simulink model "Test1"  (R2018b)
settings: Solver=VariableStepAuto  StartTime=0.0  StopTime=10.0  MaxStep=0.002  MinStep=0.001  RelTol=1e-3
undefined symbols (not defined in the file or in its folder): sigbuilder_block
settings Model: Creator=wqq  LastModifiedBy=wqq
settings SolverCC: InitialStep=0.001

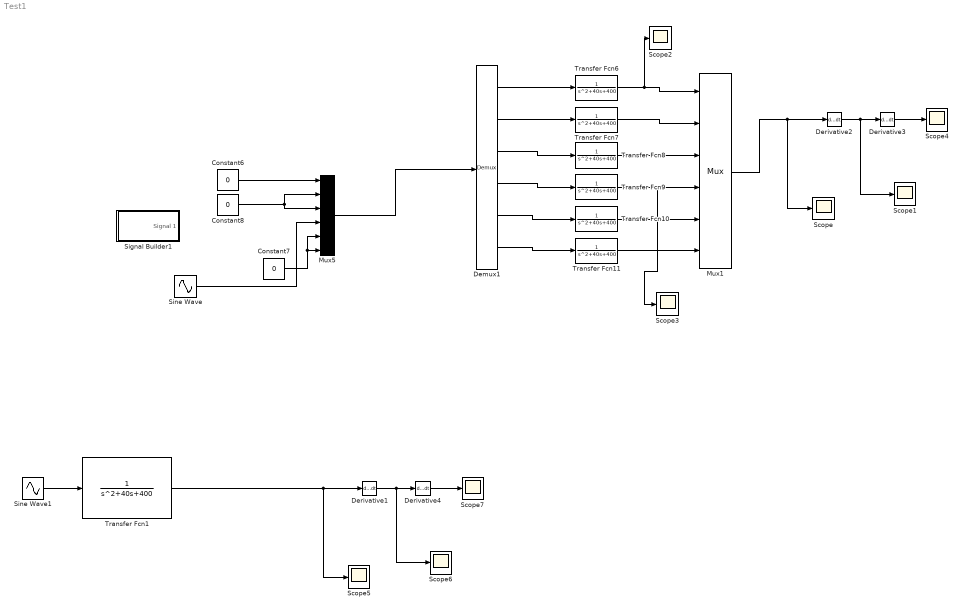
== system Test1 ==
  Constant6 : Constant  Value=0
  Constant7 : Constant  Value=0
  Constant8 : Constant  Value=0
  Demux1 : Demux  Outputs=6
  Derivative{1..4} (4 alike) : Derivative
  Mux1 : Mux  Inputs=6
  Mux5 : Mux  Inputs=6
  Scope{,1..7} (8 alike) : Scope
  Signal Builder1 : Subsystem  Tag=STV Subsys  LoadFcn=sigbuilder_block('load');  StartFcn=sigbuilder_block('start');  StopFcn=sigbuilder_block('stop');  ClipboardFcn=sigbuilder_block('clipboard');  mask(Sigbuilder block){tuvar=[0:10]}
      mask help: Simulink:masks:SigbuilderBlock_MD
      mask init:
      | if ~strcmp(get_param(bdroot(gcbh),'SimulationStatus'),'stopped') tuvar = sigbuilder_block('maskInit'); end
      settings: CopyFcn=sigbuilder_block('copy');  DeleteFcn=sigbuilder_block('delete');  ModelCloseFcn=sigbuilder_block('modelClose');  PreSaveFcn=sigbuilder_block('preSave');  PauseFcn=sigbuilder_block('pause');  ContinueFcn=sigbuilder_block('continue');  NameChangeFcn=sigbuilder_block('namechange');  OpenFcn=sigbuilder_block('open',[437.6 199.2 550.4 400 ]);  CloseFcn=sigbuilder_block('close');
      mask Display: plot(0, 0, 100, 100,[2, 2, 32, 32, 2], [68, 8, 8, 68, 68],[32, 2], [38, 38], [32, 19, 2],[53, 60, 44], [32, 17, 17, 2],[16, 16, 31, 31]);txt = getActiveGroup(gcbh);text(2, 100, txt,'verticalAlignment', 'top');
  Sine Wave : Sin  Amplitude=20  SampleTime=0
  Sine Wave1 : Sin  Amplitude=20  SampleTime=0
  Transfer Fcn{1,6..11} (7 alike) : TransferFcn  Denominator=[1 40 400]
  wires:
  Demux1/1 -> Transfer Fcn6/1
  Transfer Fcn8/1 -> Mux1/3
  Demux1/2 -> Transfer Fcn7/1
  Transfer Fcn10/1 -> Mux1/5
  Transfer Fcn7/1 -> Mux1/2
  Demux1/6 -> Transfer Fcn11/1
  Demux1/4 -> Transfer Fcn9/1
  Mux5/1 -> Demux1/1
  Transfer Fcn6/1 -> Scope2/1, Mux1/1
  Derivative2/1 -> Scope1/1, Derivative3/1
  Transfer Fcn11/1 -> Mux1/6
  Demux1/3 -> Transfer Fcn8/1
  Demux1/5 -> Transfer Fcn10/1
  Mux1/1 -> Scope/1, Derivative2/1
  Derivative3/1 -> Scope4/1
  Sine Wave/1 -> Mux5/4
  Constant6/1 -> Mux5/1
  Constant7/1 -> Mux5/5, Mux5/6
  Constant8/1 -> Mux5/2, Mux5/3
  Transfer Fcn9/1 -> Scope3/1, Mux1/4
  Sine Wave1/1 -> Transfer Fcn1/1
  Transfer Fcn1/1 -> Scope5/1, Derivative1/1
  Derivative1/1 -> Scope6/1, Derivative4/1
  Derivative4/1 -> Scope7/1

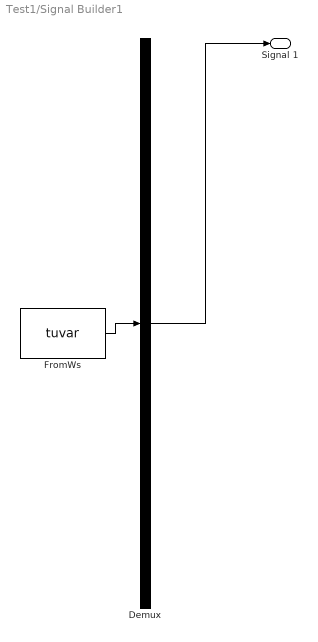
== system Test1/Signal Builder1 ==
  Demux : Demux  Tag=STV Demux  Outputs=1
  FromWs : FromWorkspace  Tag=STV FromWs  VariableName=tuvar  SampleTime=0
      SigBuilderData=|
      | common.afterFinalStr = 'Extrapolate'
      | common.sampleTime = 0
      | dataSet.timeRange = [0 10]
      | dataSet.name = 'Group 1'
      | sbobj.Groups.Name = 'Group 1'
      | sbobj.Groups.Signals.Name = 'Signal 1'
      | sbobj.Groups.Signals.XData = [0 2 4 10]
      | sbobj.Groups.Signals.YData = [0 30 0 0]
  Signal 1 : Outport  Tag=STV Outport
  wires:
  Demux/1 -> Signal 1/1
  FromWs/1 -> Demux/1
